simulink model "exer1"  (R2012b)
settings: Solver=ode45  StartTime=0.0  StopTime=10.0  RelTol=1e-3
undefined symbols (not defined in the file): alfa

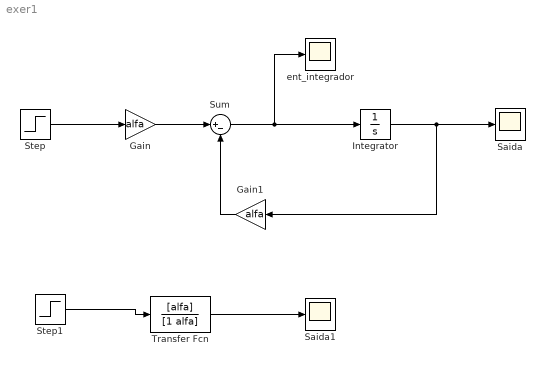
== system exer1 ==
  Gain : Gain  Gain=alfa
  Gain1 : Gain  Gain=alfa
  Integrator : Integrator
  Saida : Scope
  Saida1 : Scope
      settings: SaveName=ScopeData2
  Step : Step  SampleTime=0
  Step1 : Step  SampleTime=0
  Sum : Sum  Inputs=|+-
  Transfer Fcn : TransferFcn  Numerator=[alfa]  Denominator=[1 alfa]
  ent_integrador : Scope
  wires:
  Step/1 -> Gain/1
  Gain/1 -> Sum/1
  Sum/1 -> ent_integrador/1, Integrator/1
  Integrator/1 -> Saida/1, Gain1/1
  Gain1/1 -> Sum/2
  Step1/1 -> Transfer Fcn/1
  Transfer Fcn/1 -> Saida1/1
